simulink model "simulink_pso"  (R2017b)
settings: Solver=ode45  StartTime=0.0  StopTime=Tend  RelTol=1e-3  EnableMultiTasking=on
undefined symbols (not defined in the file): Ac_plant, Bc_plant, Cc_plant, Dc_plant, delay, F, K, pipes, ref, ref_array, ref_sampling_factor, Sat_u, Sm, Ts, variable_reference_enable, x0
libraries: dspsnks4 x2, dspsigattribs x1, dspsrcs4 x1
settings Model: Creator=rmedina  LastModifiedBy=jvalencia
settings DataIOCC: LimitDataPoints=on  SaveFormat=Array
settings OptimizationCC: LifeSpan=inf
settings DebuggingCC: SolverPrmCheckMsg=warning  SFUnexpectedBacktrackingDiag=warning  SFNoUnconditionalDefaultTransitionDiag=warning  SFExecutionAtInitializationDiag=none
settings HardwareCC: ProdBitPerPointer=32  ProdBitPerSizeT=32  ProdBitPerPtrDiffT=32  ProdLargestAtomicFloat=None  ProdIntDivRoundTo=Undefined  ProdEndianess=Unspecified  ProdWordSize=32  ProdHWDeviceType=32-bit Generic
settings ModelReferenceCC: PropagateSignalLabelsOutOfModel=off
settings CodeAppCC: StateflowObjectComments=on
settings GRTTargetCC: TargetLangStandard=C89/C90 (ANSI)  GeneratePreprocessorConditionals=Disable all
settings ConfigComp: CovMetricSettings=dw  CovHtmlReporting=on  CovSaveCumulativeToWorkspaceVar=on  CovSaveSingleToWorkspaceVar=on  CovExternalEMLEnable=off  CovSFcnEnable=off

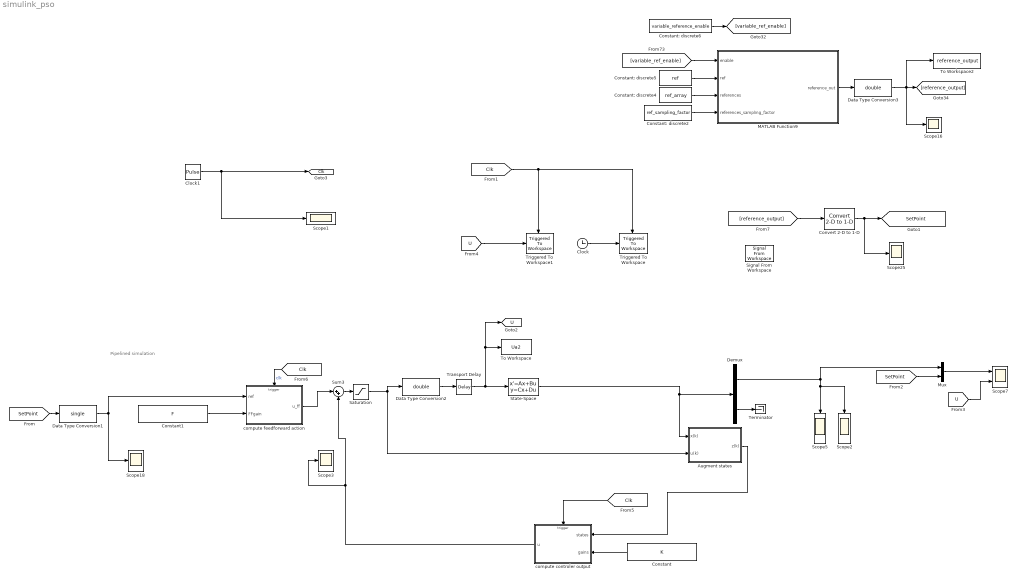
== system simulink_pso ==
  note: Pipelined simulation
  Augment states : Subsystem
  Clock : Clock
  Clock1 : DiscretePulseGenerator  PulseType=Time based  Period=Ts  PhaseDelay=1e-9
  Constant : Constant  Value=K  VectorParams1D=off
  Constant1 : Constant  Value=F  VectorParams1D=off
  Constant: discrete2 : Constant  Value=ref_sampling_factor  OutDataTypeStr=single  SampleTime=Sm
  Constant: discrete4 : Constant  Value=ref_array  OutDataTypeStr=single  SampleTime=Sm
  Constant: discrete5 : Constant  Value=ref  OutDataTypeStr=single  SampleTime=Sm
  Constant: discrete6 : Constant  Value=variable_reference_enable  SampleTime=Sm
  Convert 2-D to 1-D : dspsigattribs/Convert 2-D to 1-D
      settings: SourceProductName=DSP System Toolbox  SourceProductBaseCode=DS
  Data Type Conversion1 : DataTypeConversion  OutDataTypeStr=single
  Data Type Conversion2 : DataTypeConversion  OutDataTypeStr=double
  Data Type Conversion3 : DataTypeConversion  OutDataTypeStr=double
  Demux : Demux  Outputs=2
  MATLAB Function9 : MATLAB Function  TreatAsAtomicUnit=on
  Mux : Mux  Inputs=2
  Saturation : Saturate  UpperLimit=Sat_u(1)  LowerLimit=Sat_u(2)
  Scope{1..3,5,16,18,25} (7 alike) : Scope
  Scope7 : Scope  NumInputPorts=2
  Signal From Workspace : dspsrcs4/Signal From Workspace  X=ref  Ts=delay/8  nsamps=1  OutputAfterFinalValue=Holding final value  ignoreOrWarnInputAndFrameLengths=off  OutputFrames=on
  State-Space : StateSpace  A=Ac_plant  B=Bc_plant  C=Cc_plant  D=Dc_plant  InitialCondition=x0
  Sum3 : Sum  Inputs=|++
  Terminator : Terminator
  To Workspace : ToWorkspace  VariableName=Ua2  SaveFormat=Timeseries  SampleTime=Sm
  To Workspace2 : ToWorkspace  VariableName=reference_output  SaveFormat=Timeseries  SampleTime=Sm
  Transport Delay : TransportDelay  DelayTime=delay
  Triggered To Workspace : dspsnks4/Triggered To Workspace  TriggerType=Rising edge  VariableName=time  Buffer=1000  Save2DMode=2-D array (concatenate along first dimension)
      settings: SourceProductName=DSP System Toolbox  SourceProductBaseCode=DS  FixptAsFi=off
  Triggered To Workspace1 : dspsnks4/Triggered To Workspace  TriggerType=Rising edge  VariableName=Ua  Buffer=1000  Save2DMode=2-D array (concatenate along first dimension)
      settings: SourceProductName=DSP System Toolbox  SourceProductBaseCode=DS  FixptAsFi=off
  compute controler output : Subsystem
  compute feedforward action : Subsystem
  tag scope: Clk=global, SetPoint=global, U=global
  wires:
  Convert 2-D to 1-D/1 -> Scope25/1, [SetPoint]
  Clock1/1 -> Scope1/1, [Clk]
  compute controler output/1(u) -> Sum3/2, Scope3/1
  [SetPoint] -> Data Type Conversion1/1
  compute feedforward action/1(u_ff) -> Sum3/1
  Sum3/1 -> Saturation/1
  State-Space/1 -> Augment states/1(x(k)), Demux/1
  [Clk] -> Triggered To Workspace1/Trigger, Triggered To Workspace/Trigger
  Clock/1 -> Triggered To Workspace/1
  Saturation/1 -> Augment states/2(u(k)), Data Type Conversion2/1
  Demux/1 -> Scope2/1, Scope5/1, Mux/1
  Demux/2 -> Terminator/1
  [SetPoint] -> Mux/2
  Mux/1 -> Scope7/1
  [U] -> Scope7/2
  [U] -> Triggered To Workspace1/1
  Augment states/1(z(k)) -> compute controler output/1(states)
  Data Type Conversion1/1 -> compute feedforward action/1(ref), Scope18/1
  Data Type Conversion2/1 -> Transport Delay/1
  Constant/1 -> compute controler output/2(gains)
  [Clk] -> compute controler output/Trigger
  Constant1/1 -> compute feedforward action/2(FFgain)
  [Clk] -> compute feedforward action/Trigger  "clk"
  Transport Delay/1 -> To Workspace/1, [U], State-Space/1
  Constant: discrete4/1 -> MATLAB Function9/3(references)
  Constant: discrete5/1 -> MATLAB Function9/2(ref)
  [variable_ref_enable] -> MATLAB Function9/1(enable)
  Constant: discrete2/1 -> MATLAB Function9/4(references_sampling_factor)
  MATLAB Function9/1(reference_out) -> Data Type Conversion3/1
  Constant: discrete6/1 -> [variable_ref_enable]
  [reference_output] -> Convert 2-D to 1-D/1
  Data Type Conversion3/1 -> To Workspace2/1, Scope16/1, [reference_output]

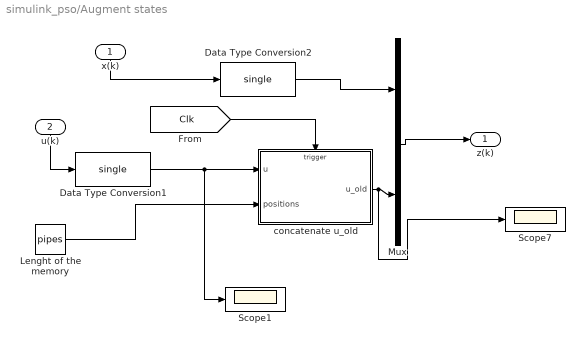
== system simulink_pso/Augment states ==
  x(k) : Inport
  u(k) : Inport  Port=2
  Data Type Conversion1 : DataTypeConversion  OutDataTypeStr=single
  Data Type Conversion2 : DataTypeConversion  OutDataTypeStr=single
  Lenght of the memory : Constant  Value=pipes
  Mux : Mux  Inputs=2
  Scope1 : Scope
  Scope7 : Scope
  concatenate u_old : Subsystem
  z(k) : Outport
  wires:
  concatenate u_old/1(u_old) -> Scope7/1, Mux/2
  Lenght of the memory/1 -> concatenate u_old/2(positions)
  [Clk] -> concatenate u_old/Trigger
  u(k)/1 -> Data Type Conversion1/1
  x(k)/1 -> Data Type Conversion2/1
  Mux/1 -> z(k)/1
  Data Type Conversion1/1 -> Scope1/1, concatenate u_old/1(u)
  Data Type Conversion2/1 -> Mux/1

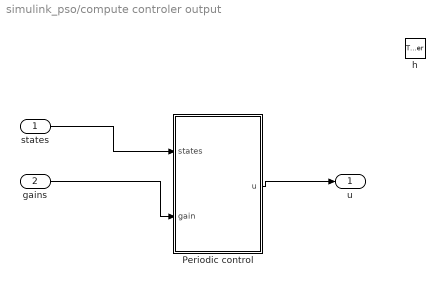
== system simulink_pso/compute controler output ==
  states : Inport
  gains : Inport  Port=2
  h : TriggerPort  VariantControl=Variant  PortDimensions=1
  Periodic control : MATLAB Function  TreatAsAtomicUnit=on
  u : Outport
  wires:
  states/1 -> Periodic control/1(states)
  Periodic control/1(u) -> u/1
  gains/1 -> Periodic control/2(gain)

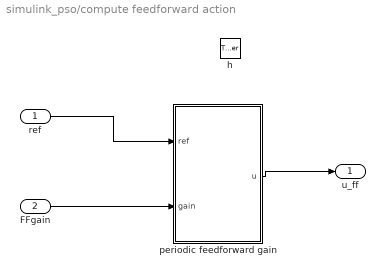
== system simulink_pso/compute feedforward action ==
  ref : Inport
  FFgain : Inport  Port=2
  h : TriggerPort  VariantControl=Variant  PortDimensions=1
  periodic feedforward gain : MATLAB Function  TreatAsAtomicUnit=on
  u_ff : Outport
  wires:
  ref/1 -> periodic feedforward gain/1(ref)
  periodic feedforward gain/1(u) -> u_ff/1
  FFgain/1 -> periodic feedforward gain/2(gain)

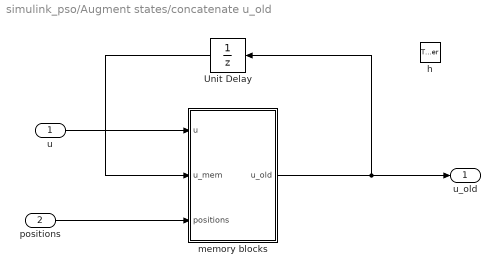
== system simulink_pso/Augment states/concatenate u_old ==
  u : Inport  LatchByDelayingOutsideSignal=on
  positions : Inport  Port=2
  h : TriggerPort  VariantControl=Variant  PortDimensions=1
  Unit Delay : UnitDelay  SampleTime=-1
  memory blocks : MATLAB Function  TreatAsAtomicUnit=on
  u_old : Outport  OutDataTypeStr=single
  wires:
  u/1 -> memory blocks/1(u)
  Unit Delay/1 -> memory blocks/2(u_mem)
  positions/1 -> memory blocks/3(positions)
  memory blocks/1(u_old) -> u_old/1, Unit Delay/1

== matlab function simulink_pso/Augment states/concatenate u_old/memory blocks ==
  data: u input single; u_mem input single size=pipes; u_old output single size=pipes; positions input [..15]
function u_old  = fcn(u,u_mem,positions)
%#codegen
assert (positions<=15);
u_old=[u_mem(2:end);u];

== matlab function simulink_pso/compute controler output/Periodic control ==
  data: u output single size=inp; states input size=states; gain input single size=[1 states]
function u  = fcn(states,gain)
%#codegen
%assert (Period<=10);
persistent K;

if (isempty(K))
    K=gain;
end


u=K*states;

== matlab function simulink_pso/compute feedforward action/periodic feedforward gain ==
  data: u output single size=inp; ref input single size=1; gain input single size=[1 1]
function u  = fcn(ref,gain)
%#codegen
%assert (Period<=10);
persistent F;

if (isempty(F))
    F=gain;
end

u=F*ref;

== matlab function simulink_pso/MATLAB Function9 ==
  data: enable input; ref input; references input; reference_out output; references_sampling_factor input
function reference_out = input_reference(enable, ref, references, references_sampling_factor)
%% VARIABLE DECLARATIONS OF COUNTERS
persistent reference_counter;
if (isempty(reference_counter)) %It does not already exist
    reference_counter = 1; % initialize with mode 1
end

persistent sampling_counter;
if (isempty(sampling_counter)) %It does not already exist
    sampling_counter = 1; % initialize with mode 1
end

%% READING INPUT VARIABLES TEMPORALLY
ref_temp        = ref;
references_temp = references;

%% OUTPUT
if enable == 1
    reference_out = single(references_temp(reference_counter));
else
    reference_out = single(ref_temp);
end

%% updating the sampling counter
if sampling_counter == references_sampling_factor
    sampling_counter = 1;
else
    sampling_counter = sampling_counter + 1;
end

%% updating the reference counter to select a different reference
if sampling_counter == 1
    if reference_counter < length(references_temp)
        reference_counter = reference_counter + 1;
    else
        reference_counter = 1;
    end
end
